simulink model "COSTEP"  (R2024b)
settings: Solver=FixedStepAuto  StartTime=0.0  StopTime=25  FixedStep=1/3600  RelTol=1e-3
model workspace (MAT data in the model file):
  AD : Simulink.Parameter (value not decoded)
  AG : Simulink.Parameter (value not decoded)
  AH : Simulink.Parameter (value not decoded)
  AV : Simulink.Parameter (value not decoded)
  AVP : Simulink.Parameter (value not decoded)
  BCHL : Simulink.Parameter (value not decoded)
  BCHV : Simulink.Parameter (value not decoded)
  BD : Simulink.Parameter (value not decoded)
  BDIST : Simulink.Parameter (value not decoded)
  BG : Simulink.Parameter (value not decoded)
  BH : Simulink.Parameter (value not decoded)
  BVP : Simulink.Parameter (value not decoded)
  CD : Simulink.Parameter (value not decoded)
  CDIST : Simulink.Parameter (value not decoded)
  CG : Simulink.Parameter (value not decoded)
  CH : Simulink.Parameter (value not decoded)
  CVP : Simulink.Parameter (value not decoded)
  DDIST : Simulink.Parameter (value not decoded)
  DIST_CONST : Simulink.Parameter (value not decoded)
  ISV : Simulink.Parameter (value not decoded)
  TLAST : Simulink.Parameter (value not decoded)
  TNEXT : Simulink.Parameter (value not decoded)
  XMW : Simulink.Parameter (value not decoded)
  XNS : Simulink.Parameter (value not decoded)
  XNS2 : Simulink.Parameter (value not decoded)
  XNS3 : Simulink.Parameter (value not decoded)
  XNSADD : Simulink.Parameter (value not decoded)
  XNSE : Simulink.Parameter (value not decoded)
symbols that are objects in the model workspace (value not decoded): AD, AG, AH, AV, AVP, BD, BG, BH, BVP, CD, CG, CH, CVP, XMW, XNS, XNS2, XNS3, XNSE
undefined symbols (not defined in the file or in its folder): magnitude, msgbox, SETPT, XMEAS, XMV
libraries: mylib x381, dspindex x31
(part 6 of 12)

== system COSTEP/Reactor/Holdup of Components in Reactor/Holdup of Vapour Components in Reactor ==
  YY(1:8) : Inport
  Bus Creator : BusCreator  Inputs=3
  Bus Selector : BusSelector  OutputSignals=YY(1),YY(2),YY(3)
  UCVR(1) Holdup of Component A (Vapour) in Reactor lb-mol : Gain
  UCVR(2) Holdup of Component B (Vapour) in Reactor lb-mol : Gain
  UCVR(3) Holdup of Component C (Vapour) in Reactor lb-mol : Gain
  UCVR : Outport  PortDimensions=3  VectorParamsAs1DForOutWhenUnconnected=off
  wires:
  UCVR(2) Holdup of Component B (Vapour) in Reactor lb-mol/1 -> Bus Creator/2  "UCVR(2)"
  Bus Selector/2 -> UCVR(2) Holdup of Component B (Vapour) in Reactor lb-mol/1  "<YY(2)>"
  Bus Selector/3 -> UCVR(3) Holdup of Component C (Vapour) in Reactor lb-mol/1  "<YY(3)>"
  UCVR(3) Holdup of Component C (Vapour) in Reactor lb-mol/1 -> Bus Creator/3  "UCVR(3)"
  UCVR(1) Holdup of Component A (Vapour) in Reactor lb-mol/1 -> Bus Creator/1  "UCVR(1)"
  Bus Creator/1 -> UCVR/1
  YY(1:8)/1 -> Bus Selector/1
  Bus Selector/1 -> UCVR(1) Holdup of Component A (Vapour) in Reactor lb-mol/1  "<YY(1)>"

== system COSTEP/Reactor/Holdup of Components in Reactor/Liquid Component Fraction in Reactor lb-mol ==
  UTLR : Inport
  UCLR : Inport  Port=2
  Bus Creator : BusCreator  Inputs=8
  Bus Selector : BusSelector  OutputSignals=UCLR(1),UCLR(2),UCLR(3),UCLR(4),UCLR(5),UCLR(6),UCLR(7),UCLR(8)
  XLR(1) : Product  Inputs=*/
  XLR(2) : Product  Inputs=*/
  XLR(3) : Product  Inputs=*/
  XLR(4) : Product  Inputs=*/
  XLR(5) : Product  Inputs=*/
  XLR(6) : Product  Inputs=*/
  XLR(7) : Product  Inputs=*/
  XLR(8) : Product  Inputs=*/
  XLR : Outport  VectorParamsAs1DForOutWhenUnconnected=off
  wires:
  XLR(5)/1 -> Bus Creator/5  "XLR(5)"
  Bus Selector/3 -> XLR(3)/1  "<UCLR(3)>"
  UTLR/1 -> XLR(8)/2, XLR(7)/2, XLR(6)/2, XLR(5)/2, XLR(4)/2, XLR(3)/2, XLR(2)/2, XLR(1)/2
  Bus Selector/7 -> XLR(7)/1  "<UCLR(7)>"
  XLR(8)/1 -> Bus Creator/8  "XLR(8)"
  XLR(7)/1 -> Bus Creator/7  "XLR(7)"
  Bus Selector/8 -> XLR(8)/1  "<UCLR(8)>"
  Bus Selector/5 -> XLR(5)/1  "<UCLR(5)>"
  Bus Selector/4 -> XLR(4)/1  "<UCLR(4)>"
  XLR(2)/1 -> Bus Creator/2  "XLR(2)"
  Bus Selector/6 -> XLR(6)/1  "<UCLR(6)>"
  XLR(3)/1 -> Bus Creator/3  "XLR(3)"
  UCLR/1 -> Bus Selector/1
  Bus Selector/1 -> XLR(1)/1  "<UCLR(1)>"
  XLR(4)/1 -> Bus Creator/4  "XLR(4)"
  Bus Selector/2 -> XLR(2)/1  "<UCLR(2)>"
  XLR(6)/1 -> Bus Creator/6  "XLR(6)"
  XLR(1)/1 -> Bus Creator/1  "XLR(1)"
  Bus Creator/1 -> XLR/1

== system COSTEP/Reactor/Holdup of Components in Reactor/Subsystem ==
  Properties of Stream 6 : Inport
  Bus Creator1 : BusCreator  Inputs=8
  Bus Selector1 : BusSelector  OutputSignals=FCM(I;6) = FCM(I;7)
  Multiport Selector : dspindex/Multiport Selector  rowsOrCols=Rows  idxCellArray={ 1,2,3,4,5,6,7,8}  idxErrMode=Clip Index
  FCM(I;7) : Outport  VectorParamsAs1DForOutWhenUnconnected=off
  wires:
  Multiport Selector/8 -> Bus Creator1/8  "FCM(8;7)"
  Multiport Selector/4 -> Bus Creator1/4  "FCM(4;7)"
  Multiport Selector/1 -> Bus Creator1/1  "FCM(1;7)"
  Bus Selector1/1 -> Multiport Selector/1  "<FCM(I;6) = FCM(I;7)>"
  Multiport Selector/6 -> Bus Creator1/6  "FCM(6;7)"
  Multiport Selector/2 -> Bus Creator1/2  "FCM(2;7)"
  Properties of Stream 6/1 -> Bus Selector1/1
  Multiport Selector/7 -> Bus Creator1/7  "FCM(7;7)"
  Multiport Selector/5 -> Bus Creator1/5  "FCM(5;7)"
  Multiport Selector/3 -> Bus Creator1/3  "FCM(3;7)"
  Bus Creator1/1 -> FCM(I;7)/1

== system COSTEP/Reactor/Holdup of Components in Reactor/Subsystem1 ==
  Bus Creator1 : BusCreator  Inputs=8
  Bus Selector2 : BusSelector  OutputSignals=signal1.FCM(I;8)
  Multiport Selector1 : dspindex/Multiport Selector  rowsOrCols=Rows  idxCellArray={ 1,2,3,4,5,6,7,8}  idxErrMode=Clip Index
  FCM(I;8) : Outport  VectorParamsAs1DForOutWhenUnconnected=off
  wires:
  Multiport Selector1/4 -> Bus Creator1/4  "FCM(4;8)"
  Multiport Selector1/5 -> Bus Creator1/5  "FCM(5;8)"
  Multiport Selector1/6 -> Bus Creator1/6  "FCM(6;8)"
  Multiport Selector1/3 -> Bus Creator1/3  "FCM(3;8)"
  Multiport Selector1/8 -> Bus Creator1/8  "FCM(8;8)"
  Bus Selector2/1 -> Multiport Selector1/1  "<FCM(I;8)>"
  Multiport Selector1/2 -> Bus Creator1/2  "FCM(2;8)"
  Multiport Selector1/7 -> Bus Creator1/7  "FCM(7;8)"
  Multiport Selector1/1 -> Bus Creator1/1  "FCM(1;8)"
  Bus Creator1/1 -> FCM(I;8)/1
  [PropertiesStream8] -> Bus Selector2/1

== system COSTEP/Reactor/Holdup of Components in Reactor/YP(1) ==
  FCM(1,7) : Inport
  CRXR(1) : Inport  Port=2
  FCM(1,8) : Inport  Port=3
  " YP(1)" : Sum  Inputs=+-+
  Bus Selector : BusSelector  OutputSignals=FCM(1;7)
  Bus Selector1 : BusSelector  OutputSignals=FCM(1;8)
  Bus Selector2 : BusSelector  OutputSignals=CRXR(1)
  Constant : Constant
  Initial state variable : mylib/Initial state variable
  Integration : mylib/Integration  SystemSampleTime=-1  VariantActivationTime=update diagram  AllowFlexibleInterface=on  Latency=0  AutoFrameSizeCalculation=off
  YY(1) : Outport  VectorParamsAs1DForOutWhenUnconnected=off
  wires:
  FCM(1,7)/1 -> Bus Selector/1
  Bus Selector/1 -> " YP(1)"/1  "<FCM(1;7)>"
  FCM(1,8)/1 -> Bus Selector1/1
  Bus Selector1/1 -> " YP(1)"/2  "<FCM(1;8)>"
  CRXR(1)/1 -> Bus Selector2/1
  Bus Selector2/1 -> " YP(1)"/3  "<CRXR(1)>"
  " YP(1)"/1 -> Integration/1
  Initial state variable/1 -> Integration/2
  Integration/1 -> YY(1)/1
  Constant/1 -> Initial state variable/1

== system COSTEP/Reactor/Holdup of Components in Reactor/YP(2) ==
  FCM(2,7) : Inport
  FCM(2,8) : Inport  Port=2
  Bus Selector : BusSelector  OutputSignals=FCM(2;7)
  Bus Selector1 : BusSelector  OutputSignals=FCM(2;8)
  Constant : Constant  Value=2
  Initial state variable : mylib/Initial state variable
  Integration : mylib/Integration  SystemSampleTime=-1  VariantActivationTime=update diagram  AllowFlexibleInterface=on  Latency=0  AutoFrameSizeCalculation=off
  "YP(2) " : Sum  Inputs=+-
  YY(2) : Outport  VectorParamsAs1DForOutWhenUnconnected=off
  wires:
  FCM(2,8)/1 -> Bus Selector1/1
  FCM(2,7)/1 -> Bus Selector/1
  Bus Selector/1 -> "YP(2) "/1  "<FCM(2;7)>"
  Bus Selector1/1 -> "YP(2) "/2  "<FCM(2;8)>"
  "YP(2) "/1 -> Integration/1
  Initial state variable/1 -> Integration/2
  Integration/1 -> YY(2)/1
  Constant/1 -> Initial state variable/1

== system COSTEP/Reactor/Holdup of Components in Reactor/YP(3) ==
  FCM(3,7) : Inport
  CRXR(3) : Inport  Port=2
  FCM(3,8) : Inport  Port=3
  " YP(3)" : Sum  Inputs=+-+
  Bus Selector : BusSelector  OutputSignals=CRXR(3)
  Bus Selector1 : BusSelector  OutputSignals=FCM(3;8)
  Bus Selector2 : BusSelector  OutputSignals=FCM(3;7)
  Constant : Constant  Value=3
  Initial state variable : mylib/Initial state variable
  Integration : mylib/Integration  SystemSampleTime=-1  VariantActivationTime=update diagram  AllowFlexibleInterface=on  Latency=0  AutoFrameSizeCalculation=off
  YY(3) : Outport  VectorParamsAs1DForOutWhenUnconnected=off
  wires:
  CRXR(3)/1 -> Bus Selector/1
  FCM(3,8)/1 -> Bus Selector1/1
  FCM(3,7)/1 -> Bus Selector2/1
  Bus Selector/1 -> " YP(3)"/3  "<CRXR(3)>"
  Bus Selector1/1 -> " YP(3)"/2  "<FCM(3;8)>"
  Bus Selector2/1 -> " YP(3)"/1  "<FCM(3;7)>"
  " YP(3)"/1 -> Integration/1
  Initial state variable/1 -> Integration/2
  Integration/1 -> YY(3)/1
  Constant/1 -> Initial state variable/1

== system COSTEP/Reactor/Holdup of Components in Reactor/YP(4) ==
  FCM(4,7) : Inport
  CRXR(4) : Inport  Port=2
  FCM(4,8) : Inport  Port=3
  " " : Sum  Inputs=+-+
  Bus Selector : BusSelector  OutputSignals=CRXR(4)
  Bus Selector1 : BusSelector  OutputSignals=FCM(4;8)
  Bus Selector2 : BusSelector  OutputSignals=FCM(4;7)
  Constant : Constant  Value=4
  Initial state variable : mylib/Initial state variable
  Integration : mylib/Integration  SystemSampleTime=-1  VariantActivationTime=update diagram  AllowFlexibleInterface=on  Latency=0  AutoFrameSizeCalculation=off
  "YY(4) " : Outport  VectorParamsAs1DForOutWhenUnconnected=off
  wires:
  CRXR(4)/1 -> Bus Selector/1
  FCM(4,8)/1 -> Bus Selector1/1
  FCM(4,7)/1 -> Bus Selector2/1
  Bus Selector/1 -> " "/3  "<CRXR(4)>"
  Bus Selector1/1 -> " "/2  "<FCM(4;8)>"
  Bus Selector2/1 -> " "/1  "<FCM(4;7)>"
  " "/1 -> Integration/1
  Initial state variable/1 -> Integration/2
  Integration/1 -> "YY(4) "/1
  Constant/1 -> Initial state variable/1

== system COSTEP/Reactor/Holdup of Components in Reactor/YP(5) ==
  FCM(5,7) : Inport
  CRXR(5) : Inport  Port=2
  FCM(5,8) : Inport  Port=3
  " " : Sum  Inputs=+-+
  Bus Selector : BusSelector  OutputSignals=CRXR(5)
  Bus Selector1 : BusSelector  OutputSignals=FCM(5;8)
  Bus Selector2 : BusSelector  OutputSignals=FCM(5;7)
  Constant : Constant  Value=5
  Initial state variable : mylib/Initial state variable
  Integration : mylib/Integration  SystemSampleTime=-1  VariantActivationTime=update diagram  AllowFlexibleInterface=on  Latency=0  AutoFrameSizeCalculation=off
  "YY(5) " : Outport  VectorParamsAs1DForOutWhenUnconnected=off
  wires:
  CRXR(5)/1 -> Bus Selector/1
  FCM(5,8)/1 -> Bus Selector1/1
  FCM(5,7)/1 -> Bus Selector2/1
  Bus Selector/1 -> " "/3  "<CRXR(5)>"
  Bus Selector1/1 -> " "/2  "<FCM(5;8)>"
  Bus Selector2/1 -> " "/1  "<FCM(5;7)>"
  " "/1 -> Integration/1
  Initial state variable/1 -> Integration/2
  Integration/1 -> "YY(5) "/1
  Constant/1 -> Initial state variable/1

== system COSTEP/Reactor/Holdup of Components in Reactor/YP(6) ==
  FCM(6,7) : Inport
  CRXR(6) : Inport  Port=2
  FCM(6,8) : Inport  Port=3
  " " : Sum  Inputs=+-+
  Bus Selector : BusSelector  OutputSignals=CRXR(6)
  Bus Selector1 : BusSelector  OutputSignals=FCM(6;8)
  Bus Selector2 : BusSelector  OutputSignals=FCM(6;7)
  Constant : Constant  Value=6
  Initial state variable : mylib/Initial state variable
  Integration : mylib/Integration  SystemSampleTime=-1  VariantActivationTime=update diagram  AllowFlexibleInterface=on  Latency=0  AutoFrameSizeCalculation=off
  "YY(6) " : Outport  VectorParamsAs1DForOutWhenUnconnected=off
  wires:
  CRXR(6)/1 -> Bus Selector/1
  FCM(6,8)/1 -> Bus Selector1/1
  FCM(6,7)/1 -> Bus Selector2/1
  Bus Selector/1 -> " "/3  "<CRXR(6)>"
  Bus Selector1/1 -> " "/2  "<FCM(6;8)>"
  Bus Selector2/1 -> " "/1  "<FCM(6;7)>"
  " "/1 -> Integration/1
  Initial state variable/1 -> Integration/2
  Integration/1 -> "YY(6) "/1
  Constant/1 -> Initial state variable/1

== system COSTEP/Reactor/Holdup of Components in Reactor/YP(7) ==
  FCM(7,7) : Inport
  CRXR(7) : Inport  Port=2
  FCM(7,8) : Inport  Port=3
  " " : Sum  Inputs=+-+
  Bus Selector : BusSelector  OutputSignals=CRXR(7)
  Bus Selector1 : BusSelector  OutputSignals=FCM(7;8)
  Bus Selector2 : BusSelector  OutputSignals=FCM(7;7)
  Constant : Constant  Value=7
  Initial state variable : mylib/Initial state variable
  Integration : mylib/Integration  SystemSampleTime=-1  VariantActivationTime=update diagram  AllowFlexibleInterface=on  Latency=0  AutoFrameSizeCalculation=off
  "YY(7) " : Outport  VectorParamsAs1DForOutWhenUnconnected=off
  wires:
  CRXR(7)/1 -> Bus Selector/1
  FCM(7,8)/1 -> Bus Selector1/1
  FCM(7,7)/1 -> Bus Selector2/1
  Bus Selector/1 -> " "/3  "<CRXR(7)>"
  Bus Selector1/1 -> " "/2  "<FCM(7;8)>"
  Bus Selector2/1 -> " "/1  "<FCM(7;7)>"
  " "/1 -> Integration/1
  Initial state variable/1 -> Integration/2
  Integration/1 -> "YY(7) "/1
  Constant/1 -> Initial state variable/1

== system COSTEP/Reactor/Holdup of Components in Reactor/YP(8) ==
  FCM(8,7) : Inport
  CRXR(8) : Inport  Port=2
  FCM(8,8) : Inport  Port=3
  " " : Sum  Inputs=+-+
  Bus Selector : BusSelector  OutputSignals=CRXR(8)
  Bus Selector1 : BusSelector  OutputSignals=FCM(8;8)
  Bus Selector2 : BusSelector  OutputSignals=FCM(8;7)
  Constant : Constant  Value=8
  Initial state variable : mylib/Initial state variable
  Integration : mylib/Integration  SystemSampleTime=-1  VariantActivationTime=update diagram  AllowFlexibleInterface=on  Latency=0  AutoFrameSizeCalculation=off
  "YY(8) " : Outport  VectorParamsAs1DForOutWhenUnconnected=off
  wires:
  CRXR(8)/1 -> Bus Selector/1
  FCM(8,8)/1 -> Bus Selector1/1
  FCM(8,7)/1 -> Bus Selector2/1
  Bus Selector/1 -> " "/3  "<CRXR(8)>"
  Bus Selector1/1 -> " "/2  "<FCM(8;8)>"
  Bus Selector2/1 -> " "/1  "<FCM(8;7)>"
  " "/1 -> Integration/1
  Initial state variable/1 -> Integration/2
  Integration/1 -> "YY(8) "/1
  Constant/1 -> Initial state variable/1

== system COSTEP/Reactor/Pressure of Reactor/Subsystem ==
  TKR : Inport
  VVR : Inport  Port=2
  UCVR : Inport  Port=3
  Bus Selector : BusSelector  OutputSignals=UCVR(1),UCVR(2),UCVR(3)
  PPR(1) Partial pressure of Component A mmHg : Product  Inputs=***/
  PPR(2) Partial pressure of Component B mmHg : Product  Inputs=***/
  PPR(3) Partial pressure of Component C mmHg : Product  Inputs=***/
  RG Universal Gas Constant ft³·mmHg/K·lb-mol : Constant  Value=998.9
  PPR(1) : Outport  VectorParamsAs1DForOutWhenUnconnected=off
  PPR(2) : Outport  Port=2  VectorParamsAs1DForOutWhenUnconnected=off
  PPR(3) : Outport  Port=3  VectorParamsAs1DForOutWhenUnconnected=off
  wires:
  Bus Selector/2 -> PPR(2) Partial pressure of Component B mmHg/1  "<UCVR(2)>"
  TKR/1 -> PPR(3) Partial pressure of Component C mmHg/3, PPR(2) Partial pressure of Component B mmHg/3, PPR(1) Partial pressure of Component A mmHg/3
  VVR/1 -> PPR(3) Partial pressure of Component C mmHg/4, PPR(2) Partial pressure of Component B mmHg/4, PPR(1) Partial pressure of Component A mmHg/4
  RG Universal Gas Constant ft³·mmHg/K·lb-mol/1 -> PPR(3) Partial pressure of Component C mmHg/2, PPR(1) Partial pressure of Component A mmHg/2, PPR(2) Partial pressure of Component B mmHg/2
  PPR(2) Partial pressure of Component B mmHg/1 -> PPR(2)/1  "PPR(2)"
  Bus Selector/1 -> PPR(1) Partial pressure of Component A mmHg/1  "<UCVR(1)>"
  Bus Selector/3 -> PPR(3) Partial pressure of Component C mmHg/1  "<UCVR(3)>"
  PPR(1) Partial pressure of Component A mmHg/1 -> PPR(1)/1  "PPR(1)"
  PPR(3) Partial pressure of Component C mmHg/1 -> PPR(3)/1  "PPR(3)"
  UCVR/1 -> Bus Selector/1

== system COSTEP/Reactor/Pressure of Reactor/VPR Vapour Pressure mmHg ==
  TCR : Inport
  AVP(I) Antoine Coefficient A ln(mmHg) : Constant  Value=AVP
  Add : Sum
  Add1 : Sum
  BVP(I) Antoine Coefficient B ln(mmHg)·°C : Constant  Value=BVP
  CVP(I) Antoine Coefficient C °C : Constant  Value=CVP
  Divide : Product  Inputs=*/
  Math Function : Math  SignedPower=on
  VPR : Outport  VectorParamsAs1DForOutWhenUnconnected=off
  wires:
  BVP(I) Antoine Coefficient B ln(mmHg)·°C/1 -> Divide/1
  CVP(I) Antoine Coefficient C °C/1 -> Add/1
  AVP(I) Antoine Coefficient A ln(mmHg)/1 -> Add1/1
  Add/1 -> Divide/2
  Divide/1 -> Add1/2
  Add1/1 -> Math Function/1
  Math Function/1 -> VPR/1
  TCR/1 -> Add/2

== system COSTEP/Reactor/Reaction Rates/Component reaction rate lb-mol//h ==
  RR : Inport
  Bus Creator : BusCreator  Inputs=7
  Subsystem : Subsystem
  Subsystem1 : Subsystem
  Subsystem2 : Subsystem
  Subsystem3 : Subsystem
  Subsystem4 : Subsystem
  Subsystem5 : Subsystem
  Subsystem6 : Subsystem
  CRXR : Outport  VectorParamsAs1DForOutWhenUnconnected=off
  wires:
  RR/1 -> Subsystem4/1(RR), Subsystem6/1(RR), Subsystem5/1(RR), Subsystem3/1(RR), Subsystem1/1(RR), Subsystem/1(RR), Subsystem2/1(RR)
  Bus Creator/1 -> CRXR/1
  Subsystem/1(CRXR(1)) -> Bus Creator/1
  Subsystem1/1(CRXR(3)) -> Bus Creator/2
  Subsystem2/1(CRXR(4)) -> Bus Creator/3
  Subsystem3/1(CRXR(5)) -> Bus Creator/4
  Subsystem4/1(CRXR(6)) -> Bus Creator/5
  Subsystem5/1(CRXR(7)) -> Bus Creator/6
  Subsystem6/1(CRXR(8)) -> Bus Creator/7

== system COSTEP/Reactor/Reaction Rates/Reaction Heat MBtu//h ==
  RR : Inport
  Bus Selector : BusSelector  OutputSignals=RR(1),RR(2)
  HTR(1) Heat of Reaction 1 MBtu/lb-mol : Constant  Value=0.06899381054
  HTR(2) Heat of reaction 2 MBtu/lb-mol : Constant  Value=0.05
  Product : Product
  Product1 : Product
  RH Total reaction heat MBtu/h : Sum
  RH : Outport  VectorParamsAs1DForOutWhenUnconnected=off
  wires:
  HTR(2) Heat of reaction 2 MBtu/lb-mol/1 -> Product1/2
  Product/1 -> RH Total reaction heat MBtu/h/1
  Product1/1 -> RH Total reaction heat MBtu/h/2
  HTR(1) Heat of Reaction 1 MBtu/lb-mol/1 -> Product/2
  RH Total reaction heat MBtu/h/1 -> RH/1
  RR/1 -> Bus Selector/1
  Bus Selector/1 -> Product/1  "<RR(1)>"
  Bus Selector/2 -> Product1/1  "<RR(2)>"

== system COSTEP/Reactor/Reaction Rates/Reaction rates lb-mol//h ==
  TKR : Inport
  PPR : Inport  Port=2
  VVR : Inport  Port=3
  " Reaction rate of reaction 4 lb-mol/ft3·h    " : Subsystem
  Bus Creator : BusCreator  Inputs=4
  Product{,1..3} (4 alike) : Product
  Reaction rate of reaction 1 lb-mol/ft3·h : Subsystem
  Reaction rate of reaction 2 lb-mol/ft3·h : Subsystem
  "Reaction rate of reaction 3 lb-mol/ft3·h  " : Subsystem
  RR : Outport  VectorParamsAs1DForOutWhenUnconnected=off
  wires:
  TKR/1 -> Reaction rate of reaction 1 lb-mol/ft3·h/2(TKR), " Reaction rate of reaction 4 lb-mol/ft3·h    "/2(TKR), "Reaction rate of reaction 3 lb-mol/ft3·h  "/2(TKR), Reaction rate of reaction 2 lb-mol/ft3·h/2(TKR)
  PPR/1 -> Reaction rate of reaction 1 lb-mol/ft3·h/1(PPR), " Reaction rate of reaction 4 lb-mol/ft3·h    "/1(PPR), "Reaction rate of reaction 3 lb-mol/ft3·h  "/1(PPR), Reaction rate of reaction 2 lb-mol/ft3·h/1(PPR)
  Bus Creator/1 -> RR/1
  Reaction rate of reaction 1 lb-mol/ft3·h/1(RR(1)) -> Product/1  "RR(1)"
  VVR/1 -> Product/2, Product3/2, Product2/2, Product1/2
  Product/1 -> Bus Creator/1  "RR(1)"
  Reaction rate of reaction 2 lb-mol/ft3·h/1(RR(2)) -> Product1/1  "RR(2)"
  Product1/1 -> Bus Creator/2  "RR(2)"
  "Reaction rate of reaction 3 lb-mol/ft3·h  "/1(RR(3)) -> Product2/1  "RR(3)"
  Product2/1 -> Bus Creator/3  "RR(3)"
  " Reaction rate of reaction 4 lb-mol/ft3·h    "/1(RR(4)) -> Product3/1  "RR(4)"
  Product3/1 -> Bus Creator/4  "RR(4)"

== system COSTEP/Reactor/Reactor Heat exchanger/Position of Valve 10 % ==
  Bus Selector : BusSelector  OutputSignals=XMV(10)
  Bus Selector1 : BusSelector  OutputSignals=IDV(14)
  Constant : Constant  Value=48
  Control valve : mylib/Control valve  SystemSampleTime=-1  VariantActivationTime=update diagram  AllowFlexibleInterface=on  Latency=0  AutoFrameSizeCalculation=off
  Divide : Product  Inputs=*/
  Initial state variable : mylib/Initial state variable
  Integration : mylib/Integration  SystemSampleTime=-1  VariantActivationTime=update diagram  AllowFlexibleInterface=on  Latency=0  AutoFrameSizeCalculation=off
  Subtract : Sum  Inputs=+-
  VTAU(10) : Constant  Value=5/3600
  "YY(48) " : Outport  PortDimensions=1  VectorParamsAs1DForOutWhenUnconnected=off
  wires:
  Subtract/1 -> Divide/1
  Control valve/1 -> Subtract/1
  VTAU(10)/1 -> Divide/2
  Divide/1 -> Integration/1
  [XMV] -> Bus Selector/1
  Bus Selector/1 -> Control valve/1  "<XMV(10)>"
  [IDV] -> Bus Selector1/1
  Bus Selector1/1 -> Control valve/2  "<IDV(14)>"
  Initial state variable/1 -> Integration/2
  Integration/1 -> Subtract/2, "YY(48) "/1
  Constant/1 -> Initial state variable/1

== system COSTEP/Reactor/Reactor Heat exchanger/Position of Valve 12 % ==
  Bus Selector : BusSelector  OutputSignals=XMV(12)
  Constant : Constant  Value=50
  Control valve : Subsystem
  Divide : Product  Inputs=*/
  Initial state variable : mylib/Initial state variable
  Integration : mylib/Integration  SystemSampleTime=-1  VariantActivationTime=update diagram  AllowFlexibleInterface=on  Latency=0  AutoFrameSizeCalculation=off
  Subtract : Sum  Inputs=+-
  VTAU(12) : Constant  Value=5/3600
  "YY(50) " : Outport  PortDimensions=1  VectorParamsAs1DForOutWhenUnconnected=off
  wires:
  Integration/1 -> "YY(50) "/1, Subtract/2  "VPOS(12)"
  Subtract/1 -> Divide/1
  Control valve/1(VCV(12)) -> Subtract/1
  VTAU(12)/1 -> Divide/2
  Divide/1 -> Integration/1
  Initial state variable/1 -> Integration/2
  [XMV] -> Bus Selector/1
  Bus Selector/1 -> Control valve/1(XMV(12))  "<XMV(12)>"
  Constant/1 -> Initial state variable/1

== system COSTEP/Reactor/Reactor Heat exchanger/Reactor Heat exchanger ==
  VLR : Inport
  VPOS(10) : Inport  Port=2
  VRNG(10) : Inport  Port=3
  VPOS(12) : Inport  Port=4
  TCR : Inport  Port=5
  AGSP Agitation speed : Subsystem
  Cooling water outlet temperature : Subsystem
  FWR Flow of cooling water to reactor gallons per minute : Subsystem
  Subsystem : Subsystem
  Subsystem2 : Subsystem
  Subsystem3 : Subsystem
  "QUR " : Outport  PortDimensions=1  VectorParamsAs1DForOutWhenUnconnected=off
  tag scope: FWR=global
  wires:
  VRNG(10)/1 -> FWR Flow of cooling water to reactor gallons per minute/2(VRNG(10))
  VLR/1 -> Subsystem/1(VLR)
  VPOS(10)/1 -> FWR Flow of cooling water to reactor gallons per minute/1(VPOS(10))
  VPOS(12)/1 -> AGSP Agitation speed/1(VPOS(12))
  FWR Flow of cooling water to reactor gallons per minute/1(FWR) -> [FWR], Cooling water outlet temperature/1(FWR)
  Subsystem/1("UARLEV ") -> Subsystem2/1(UARLEV)
  AGSP Agitation speed/1(AGSP) -> Subsystem2/2(AGSP)
  Subsystem3/1("QUR ") -> Cooling water outlet temperature/2(QUR), "QUR "/1
  Subsystem2/1("UAR ") -> Subsystem3/1(UAR)
  Cooling water outlet temperature/1("YY(37) ") -> Subsystem3/2(TWR)
  TCR/1 -> Subsystem3/3(TCR)

== system COSTEP/Reactor/Reactor Heat exchanger/VRNG(10) Max flow of water through valve Gallons per minute ==
  Bus Selector : BusSelector  OutputSignals=signal3.TESUB8(19)
  VRNG(10) : Outport  PortDimensions=1  VectorParamsAs1DForOutWhenUnconnected=off
  wires:
  [TESUB8] -> Bus Selector/1
  Bus Selector/1 -> VRNG(10)/1  "<TESUB8(19)>"

== system COSTEP/Reactor/Stream 8/HST(8) Molar Enthalpy of Stream 8 MBtu//lb-mol ==
  ITY : Inport
  T : Inport  Port=2
  XST(I,I) : Inport  Port=3
  "Enthalpy of Stream " : mylib/Enthalpy of Stream   SystemSampleTime=-1  VariantActivationTime=update diagram  AllowFlexibleInterface=on  Latency=0  AutoFrameSizeCalculation=off
  "H " : Outport  VectorParamsAs1DForOutWhenUnconnected=off
  wires:
  ITY/1 -> "Enthalpy of Stream "/1
  T/1 -> "Enthalpy of Stream "/2
  XST(I,I)/1 -> "Enthalpy of Stream "/3
  "Enthalpy of Stream "/1 -> "H "/1

== system COSTEP/Reactor/Stream 8/Subsystem ==
  Abs : Abs  SaturateOnIntegerOverflow=off
  Bus Selector : BusSelector  OutputSignals=signal2.TESUB8(12)
  Constant : Constant  Value=0.0
  Constant1 : Constant  Value=4574.21
  Constant2 : Constant
  Constant3 : Constant  Value=0.25
  DLP : Sum  Inputs=+-
  DLP Pressure drop between separator and reactor : Merge
  FLMS : Product  Inputs=3
  If : If  IfExpression=u1 < 0
  If Action Subsystem : Subsystem  TreatAsAtomicUnit=on
  If Action Subsystem1 : Subsystem  TreatAsAtomicUnit=on
  Product : Product
  Sqrt : Sqrt
  Subtract : Sum  Inputs=+-
  "FLMS " : Outport  VectorParamsAs1DForOutWhenUnconnected=off
  wires:
  [PTS] -> DLP/2
  If Action Subsystem/1(Out1) -> DLP Pressure drop between separator and reactor/1
  Constant2/1 -> Subtract/1
  DLP/1 -> If/1, If Action Subsystem1/1(In1)
  DLP Pressure drop between separator and reactor/1 -> Abs/1
  If Action Subsystem1/1(Out1) -> DLP Pressure drop between separator and reactor/2
  If/1 -> If Action Subsystem/Action
  Sqrt/1 -> FLMS/2
  [PTR] -> DLP/1
  Abs/1 -> Sqrt/1
  Constant3/1 -> Product/1
  Constant1/1 -> FLMS/1
  [TESUB8] -> Bus Selector/1
  Subtract/1 -> FLMS/3
  Bus Selector/1 -> Product/2  "<TESUB8(12)>"
  If/2 -> If Action Subsystem1/Action
  Product/1 -> Subtract/2
  Constant/1 -> If Action Subsystem/1(In1)
  FLMS/1 -> "FLMS "/1

== system COSTEP/Reactor/Stream 8/XMWS(8) Molecular weight of Stream 8 lb//lb-mol ==
  XST(I,8) : Inport
  Product : Product
  Sum of Elements : Sum  Inputs=+
  "XMW(I) Molecular weight of components lb/lb-mol " : Constant  Value=[2;25.4;28;32;46;48;62;76]
  XMWS(8) : Outport  VectorParamsAs1DForOutWhenUnconnected=off
  wires:
  Sum of Elements/1 -> XMWS(8)/1
  Product/1 -> Sum of Elements/1
  XST(I,8)/1 -> Product/1
  "XMW(I) Molecular weight of components lb/lb-mol "/1 -> Product/2

== system COSTEP/Reactor/Volume of Reactor/DLR Molar Density of Liquids in Reactor lb-mol//ft³     ==
  XLR : Inport
  TCR : Inport  Port=2
  "DLR Molar Density of Liquids in Reactor lb-mol/ft³ " : Subsystem
  "DLR " : Outport  VectorParamsAs1DForOutWhenUnconnected=off
  wires:
  "DLR Molar Density of Liquids in Reactor lb-mol/ft³ "/1("R ") -> "DLR "/1
  TCR/1 -> "DLR Molar Density of Liquids in Reactor lb-mol/ft³ "/2(T)
  XLR/1 -> "DLR Molar Density of Liquids in Reactor lb-mol/ft³ "/1(X)

== system COSTEP/Separator/Holdup of Components in Separator/Holdup of Liquid Components in Separator ==
  YY(10:17) : Inport
  Bus Creator : BusCreator  Inputs=8
  Bus Selector : BusSelector  OutputSignals=YY(13),YY(14),YY(15),YY(16),YY(17)
  UCLS(1) Holdup of Component A (Liquid) in Separator lb-mol : Constant  Value=0
  UCLS(2) Holdup of Component B (Liquid) in Separator lb-mol : Constant  Value=0
  UCLS(4) Holdup of Component D (Liquid) in Separator lb-mol : Gain
  UCLS(5) Holdup of Component E (Liquid) in Separator lb-mol : Gain
  UCLS(6) Holdup of Component F (Liquid) in Separator lb-mol : Gain
  UCLS(7) Holdup of Component G (Liquid) in Separator lb-mol : Gain
  UCLS(8) Holdup of Component H (Liquid) in Separator lb-mol : Gain
  UCLS3) Holdup of Component C (Liquid) in Separator lb-mol : Constant  Value=0
  UCLS : Outport  VectorParamsAs1DForOutWhenUnconnected=off
  wires:
  UCLS(2) Holdup of Component B (Liquid) in Separator lb-mol/1 -> Bus Creator/2  "UCLS(2)"
  UCLS(8) Holdup of Component H (Liquid) in Separator lb-mol/1 -> Bus Creator/8  "UCLS(8)"
  UCLS(1) Holdup of Component A (Liquid) in Separator lb-mol/1 -> Bus Creator/1  "UCLS(1)"
  UCLS(5) Holdup of Component E (Liquid) in Separator lb-mol/1 -> Bus Creator/5  "UCLS(5)"
  UCLS(4) Holdup of Component D (Liquid) in Separator lb-mol/1 -> Bus Creator/4  "UCLS(4)"
  UCLS3) Holdup of Component C (Liquid) in Separator lb-mol/1 -> Bus Creator/3  "UCLS(3)"
  UCLS(6) Holdup of Component F (Liquid) in Separator lb-mol/1 -> Bus Creator/6  "UCLS(6)"
  UCLS(7) Holdup of Component G (Liquid) in Separator lb-mol/1 -> Bus Creator/7  "UCLS(7)"
  YY(10:17)/1 -> Bus Selector/1
  Bus Creator/1 -> UCLS/1
  Bus Selector/1 -> UCLS(4) Holdup of Component D (Liquid) in Separator lb-mol/1  "<YY(13)>"
  Bus Selector/2 -> UCLS(5) Holdup of Component E (Liquid) in Separator lb-mol/1  "<YY(14)>"
  Bus Selector/3 -> UCLS(6) Holdup of Component F (Liquid) in Separator lb-mol/1  "<YY(15)>"
  Bus Selector/4 -> UCLS(7) Holdup of Component G (Liquid) in Separator lb-mol/1  "<YY(16)>"
  Bus Selector/5 -> UCLS(8) Holdup of Component H (Liquid) in Separator lb-mol/1  "<YY(17)>"

== system COSTEP/Separator/Holdup of Components in Separator/Holdup of Vapour Components in Separator ==
  YY(10:17) : Inport
  Bus Creator : BusCreator  Inputs=3
  Bus Selector : BusSelector  OutputSignals=YY(10),YY(11),YY(12)
  UCVS(1) Holdup of Component A (Vapour) in Separator lb-mol : Gain
  UCVS(2) Holdup of Component B (Vapour) in Separator lb-mol : Gain
  UCVS(3) Holdup of Component C (Vapour) in Separator lb-mol : Gain
  UCVS : Outport  VectorParamsAs1DForOutWhenUnconnected=off
  wires:
  UCVS(1) Holdup of Component A (Vapour) in Separator lb-mol/1 -> Bus Creator/1  "UCVS(1)"
  Bus Selector/3 -> UCVS(3) Holdup of Component C (Vapour) in Separator lb-mol/1  "<YY(12)>"
  UCVS(2) Holdup of Component B (Vapour) in Separator lb-mol/1 -> Bus Creator/2  "UCVS(2)"
  UCVS(3) Holdup of Component C (Vapour) in Separator lb-mol/1 -> Bus Creator/3  "UCVS(3)"
  Bus Creator/1 -> UCVS/1
  YY(10:17)/1 -> Bus Selector/1
  Bus Selector/1 -> UCVS(1) Holdup of Component A (Vapour) in Separator lb-mol/1  "<YY(10)>"
  Bus Selector/2 -> UCVS(2) Holdup of Component B (Vapour) in Separator lb-mol/1  "<YY(11)>"

== system COSTEP/Separator/Holdup of Components in Separator/Liquid Component Fraction in Separator ==
  UTLS : Inport
  UCLS : Inport  Port=2
  Bus Creator : BusCreator  Inputs=8
  Bus Selector : BusSelector  OutputSignals=UCLS(1),UCLS(2),UCLS(3),UCLS(4),UCLS(5),UCLS(6),UCLS(7),UCLS(8)
  XLS(1) : Product  Inputs=*/
  XLS(2) : Product  Inputs=*/
  XLS(3) : Product  Inputs=*/
  XLS(4) : Product  Inputs=*/
  XLS(5) : Product  Inputs=*/
  XLS(6) : Product  Inputs=*/
  XLS(7) : Product  Inputs=*/
  XLS(8) : Product  Inputs=*/
  XLS : Outport  VectorParamsAs1DForOutWhenUnconnected=off
  wires:
  Bus Selector/1 -> XLS(1)/1  "<UCLS(1)>"
  XLS(2)/1 -> Bus Creator/2  "XLS(2)"
  Bus Selector/7 -> XLS(7)/1  "<UCLS(7)>"
  XLS(3)/1 -> Bus Creator/3  "XLS(3)"
  Bus Selector/8 -> XLS(8)/1  "<UCLS(8)>"
  Bus Selector/3 -> XLS(3)/1  "<UCLS(3)>"
  XLS(7)/1 -> Bus Creator/7  "XLS(7)"
  XLS(1)/1 -> Bus Creator/1  "XLS(1)"
  Bus Selector/2 -> XLS(2)/1  "<UCLS(2)>"
  Bus Selector/5 -> XLS(5)/1  "<UCLS(5)>"
  Bus Selector/4 -> XLS(4)/1  "<UCLS(4)>"
  XLS(6)/1 -> Bus Creator/6  "XLS(6)"
  XLS(4)/1 -> Bus Creator/4  "XLS(4)"
  XLS(5)/1 -> Bus Creator/5  "XLS(5)"
  XLS(8)/1 -> Bus Creator/8  "XLS(8)"
  Bus Selector/6 -> XLS(6)/1  "<UCLS(6)>"
  Bus Creator/1 -> XLS/1
  UTLS/1 -> XLS(8)/2, XLS(7)/2, XLS(6)/2, XLS(5)/2, XLS(4)/2, XLS(3)/2, XLS(2)/2, XLS(1)/2
  UCLS/1 -> Bus Selector/1

== system COSTEP/Separator/Holdup of Components in Separator/Subsystem ==
  Properties of Stream 8 : Inport
  Bus Creator : BusCreator  Inputs=8
  Bus Selector : BusSelector  OutputSignals=FCM(I;8)
  FCM(1,8) : Gain
  FCM(2,8) : Gain
  FCM(3,8) : Gain
  FCM(4,8) : Gain
  FCM(5,8) : Gain
  FCM(6,8) : Gain
  FCM(7,8) : Gain
  FCM(8,8) : Gain
  Multiport Selector : dspindex/Multiport Selector  rowsOrCols=Rows  idxCellArray={ 1,2,3,4,5,6,7,8}  idxErrMode=Clip Index
  FCM(I;8) : Outport  VectorParamsAs1DForOutWhenUnconnected=off
  wires:
  Multiport Selector/3 -> FCM(3,8)/1
  Multiport Selector/6 -> FCM(6,8)/1
  Multiport Selector/8 -> FCM(8,8)/1
  Multiport Selector/2 -> FCM(2,8)/1
  Multiport Selector/7 -> FCM(7,8)/1
  Properties of Stream 8/1 -> Bus Selector/1
  Multiport Selector/4 -> FCM(4,8)/1
  Multiport Selector/1 -> FCM(1,8)/1
  Multiport Selector/5 -> FCM(5,8)/1
  Bus Selector/1 -> Multiport Selector/1  "<FCM(I;8)>"
  FCM(1,8)/1 -> Bus Creator/1  "FCM(1;8)"
  FCM(2,8)/1 -> Bus Creator/2  "FCM(2;8)"
  FCM(3,8)/1 -> Bus Creator/3  "FCM(3;8)"
  FCM(4,8)/1 -> Bus Creator/4  "FCM(4;8)"
  FCM(5,8)/1 -> Bus Creator/5  "FCM(5;8)"
  FCM(6,8)/1 -> Bus Creator/6  "FCM(6;8)"
  FCM(7,8)/1 -> Bus Creator/7  "FCM(7;8)"
  FCM(8,8)/1 -> Bus Creator/8  "FCM(8;8)"
  Bus Creator/1 -> FCM(I;8)/1

== system COSTEP/Separator/Holdup of Components in Separator/Subsystem1 ==
  Bus Creator : BusCreator  Inputs=8
  Bus Selector1 : BusSelector  OutputSignals=signal2.FCM(I;9)
  FCM(1,9) : Gain
  FCM(2,9) : Gain
  FCM(3,9) : Gain
  FCM(4,9) : Gain
  FCM(5,9) : Gain
  FCM(6,9) : Gain
  FCM(7,9) : Gain
  FCM(8,9) : Gain
  Multiport Selector1 : dspindex/Multiport Selector  rowsOrCols=Rows  idxCellArray={ 1,2,3,4,5,6,7,8}  idxErrMode=Clip Index
  FCM(I;9) : Outport  VectorParamsAs1DForOutWhenUnconnected=off
  wires:
  [PropertiesStream9] -> Bus Selector1/1
  Multiport Selector1/4 -> FCM(4,9)/1
  Bus Selector1/1 -> Multiport Selector1/1  "<FCM(I;9)>"
  Multiport Selector1/7 -> FCM(7,9)/1
  Multiport Selector1/3 -> FCM(3,9)/1
  Multiport Selector1/8 -> FCM(8,9)/1
  Multiport Selector1/6 -> FCM(6,9)/1
  Multiport Selector1/5 -> FCM(5,9)/1
  Multiport Selector1/2 -> FCM(2,9)/1
  Multiport Selector1/1 -> FCM(1,9)/1
  FCM(1,9)/1 -> Bus Creator/1  "FCM(1;9)"
  FCM(2,9)/1 -> Bus Creator/2  "FCM(2;9)"
  FCM(3,9)/1 -> Bus Creator/3  "FCM(3;9)"
  FCM(4,9)/1 -> Bus Creator/4  "FCM(4;9)"
  FCM(5,9)/1 -> Bus Creator/5  "FCM(5;9)"
  FCM(7,9)/1 -> Bus Creator/7  "FCM(7;9)"
  FCM(8,9)/1 -> Bus Creator/8  "FCM(8;9)"
  FCM(6,9)/1 -> Bus Creator/6  "FCM(6;9)"
  Bus Creator/1 -> FCM(I;9)/1

== system COSTEP/Separator/Holdup of Components in Separator/Subsystem2 ==
  Bus Creator : BusCreator  Inputs=8
  Bus Selector2 : BusSelector  OutputSignals=signal1.FCM(I;10)
  FCM(1,10) : Gain
  FCM(2,10) : Gain
  FCM(3,10) : Gain
  FCM(4,10) : Gain
  FCM(5,10) : Gain
  FCM(6,10) : Gain
  FCM(7,10) : Gain
  FCM(8,10) : Gain
  Multiport Selector2 : dspindex/Multiport Selector  rowsOrCols=Rows  idxCellArray={ 1,2,3,4,5,6,7,8}  idxErrMode=Clip Index
  FCM(I;10) : Outport  VectorParamsAs1DForOutWhenUnconnected=off
  wires:
  [PropertiesStream10] -> Bus Selector2/1
  FCM(4,10)/1 -> Bus Creator/4  "FCM(4;10)"
  Multiport Selector2/5 -> FCM(5,10)/1
  Multiport Selector2/4 -> FCM(4,10)/1
  FCM(2,10)/1 -> Bus Creator/2  "FCM(2;10)"
  Multiport Selector2/8 -> FCM(8,10)/1
  Multiport Selector2/7 -> FCM(7,10)/1
  FCM(8,10)/1 -> Bus Creator/8  "FCM(8;10)"
  Multiport Selector2/2 -> FCM(2,10)/1
  Multiport Selector2/3 -> FCM(3,10)/1
  Multiport Selector2/1 -> FCM(1,10)/1
  Bus Selector2/1 -> Multiport Selector2/1  "<FCM(I;10)>"
  Multiport Selector2/6 -> FCM(6,10)/1
  FCM(5,10)/1 -> Bus Creator/5  "FCM(5;10)"
  FCM(3,10)/1 -> Bus Creator/3  "FCM(3;10)"
  FCM(1,10)/1 -> Bus Creator/1  "FCM(1;10)"
  FCM(6,10)/1 -> Bus Creator/6  "FCM(6;10)"
  FCM(7,10)/1 -> Bus Creator/7  "FCM(7;10)"
  Bus Creator/1 -> FCM(I;10)/1

== system COSTEP/Separator/Holdup of Components in Separator/Subsystem3 ==
  Bus Creator : BusCreator  Inputs=8
  Bus Selector3 : BusSelector  OutputSignals=signal1.FCM(I;11)
  FCM(1,11) : Gain
  FCM(2,11) : Gain
  FCM(3,11) : Gain
  FCM(4,11) : Gain
  FCM(5,11) : Gain
  FCM(6,11) : Gain
  FCM(7,11) : Gain
  FCM(8,11) : Gain
  Multiport Selector3 : dspindex/Multiport Selector  rowsOrCols=Rows  idxCellArray={1,2,3,4,5,6,7,8}  idxErrMode=Clip Index
  FCM(I;11) : Outport  VectorParamsAs1DForOutWhenUnconnected=off
  wires:
  Multiport Selector3/3 -> FCM(3,11)/1
  Multiport Selector3/2 -> FCM(2,11)/1
  Multiport Selector3/5 -> FCM(5,11)/1
  Multiport Selector3/8 -> FCM(8,11)/1
  Bus Selector3/1 -> Multiport Selector3/1  "<FCM(I;11)>"
  Multiport Selector3/7 -> FCM(7,11)/1
  Multiport Selector3/6 -> FCM(6,11)/1
  Multiport Selector3/1 -> FCM(1,11)/1
  Multiport Selector3/4 -> FCM(4,11)/1
  [PropertiesStream11] -> Bus Selector3/1
  FCM(5,11)/1 -> Bus Creator/5  "FCM(5;11)"
  FCM(8,11)/1 -> Bus Creator/8  "FCM(8;11)"
  FCM(7,11)/1 -> Bus Creator/7  "FCM(7;11)"
  FCM(6,11)/1 -> Bus Creator/6  "FCM(6;11)"
  FCM(2,11)/1 -> Bus Creator/2  "FCM(2;11)"
  FCM(3,11)/1 -> Bus Creator/3  "FCM(3;11)"
  FCM(4,11)/1 -> Bus Creator/4  "FCM(4;11)"
  FCM(1,11)/1 -> Bus Creator/1  "FCM(1;11)"
  Bus Creator/1 -> FCM(I;11)/1

== system COSTEP/Separator/Holdup of Components in Separator/YP(10) ==
  FCM(1,8) : Inport
  FCM(1,9) : Inport  Port=2
  FCM(1,10) : Inport  Port=3
  FCM(1,11) : Inport  Port=4
  " " : Sum  Inputs=+---
  Bus Selector : BusSelector  OutputSignals=FCM(1;8)
  Bus Selector1 : BusSelector  OutputSignals=FCM(1;9)
  Bus Selector2 : BusSelector  OutputSignals=FCM(1;10)
  Bus Selector3 : BusSelector  OutputSignals=FCM(1;11)
  Constant : Constant  Value=10
  Initial state variable : mylib/Initial state variable
  Integration : mylib/Integration  SystemSampleTime=-1  VariantActivationTime=update diagram  AllowFlexibleInterface=on  Latency=0  AutoFrameSizeCalculation=off
  YY(10) : Outport  VectorParamsAs1DForOutWhenUnconnected=off
  wires:
  Initial state variable/1 -> Integration/2
  FCM(1,10)/1 -> Bus Selector2/1
  FCM(1,9)/1 -> Bus Selector1/1
  FCM(1,8)/1 -> Bus Selector/1
  " "/1 -> Integration/1
  Integration/1 -> YY(10)/1
  FCM(1,11)/1 -> Bus Selector3/1
  Bus Selector/1 -> " "/1  "<FCM(1;8)>"
  Bus Selector1/1 -> " "/2  "<FCM(1;9)>"
  Bus Selector2/1 -> " "/3  "<FCM(1;10)>"
  Bus Selector3/1 -> " "/4  "<FCM(1;11)>"
  Constant/1 -> Initial state variable/1

== system COSTEP/Separator/Holdup of Components in Separator/YP(11) ==
  FCM(2,8) : Inport
  FCM(2,9) : Inport  Port=2
  FCM(2,10) : Inport  Port=3
  FCM(2,11) : Inport  Port=4
  " " : Sum  Inputs=+---
  Bus Selector : BusSelector  OutputSignals=FCM(2;8)
  Bus Selector1 : BusSelector  OutputSignals=FCM(2;9)
  Bus Selector2 : BusSelector  OutputSignals=FCM(2;10)
  Bus Selector3 : BusSelector  OutputSignals=FCM(2;11)
  Constant : Constant  Value=11
  Initial state variable : mylib/Initial state variable
  Integration : mylib/Integration  SystemSampleTime=-1  VariantActivationTime=update diagram  AllowFlexibleInterface=on  Latency=0  AutoFrameSizeCalculation=off
  YY(11) : Outport  VectorParamsAs1DForOutWhenUnconnected=off
  wires:
  Integration/1 -> YY(11)/1
  FCM(2,8)/1 -> Bus Selector/1
  FCM(2,9)/1 -> Bus Selector1/1
  FCM(2,10)/1 -> Bus Selector2/1
  FCM(2,11)/1 -> Bus Selector3/1
  Initial state variable/1 -> Integration/2
  " "/1 -> Integration/1
  Bus Selector/1 -> " "/1  "<FCM(2;8)>"
  Bus Selector1/1 -> " "/2  "<FCM(2;9)>"
  Bus Selector2/1 -> " "/3  "<FCM(2;10)>"
  Bus Selector3/1 -> " "/4  "<FCM(2;11)>"
  Constant/1 -> Initial state variable/1

== system COSTEP/Separator/Holdup of Components in Separator/YP(12) ==
  FCM(3,8) : Inport
  FCM(3,9) : Inport  Port=2
  FCM(3,10) : Inport  Port=3
  FCM(3,11) : Inport  Port=4
  " " : Sum  Inputs=+---
  Bus Selector : BusSelector  OutputSignals=FCM(3;11)
  Bus Selector1 : BusSelector  OutputSignals=FCM(3;10)
  Bus Selector2 : BusSelector  OutputSignals=FCM(3;9)
  Bus Selector3 : BusSelector  OutputSignals=FCM(3;8)
  Constant : Constant  Value=12
  Initial state variable : mylib/Initial state variable
  Integration : mylib/Integration  SystemSampleTime=-1  VariantActivationTime=update diagram  AllowFlexibleInterface=on  Latency=0  AutoFrameSizeCalculation=off
  YY(12) : Outport  VectorParamsAs1DForOutWhenUnconnected=off
  wires:
  Integration/1 -> YY(12)/1
  FCM(3,8)/1 -> Bus Selector3/1
  FCM(3,9)/1 -> Bus Selector2/1
  FCM(3,10)/1 -> Bus Selector1/1
  FCM(3,11)/1 -> Bus Selector/1
  " "/1 -> Integration/1
  Initial state variable/1 -> Integration/2
  Bus Selector3/1 -> " "/1  "<FCM(3;8)>"
  Bus Selector2/1 -> " "/2  "<FCM(3;9)>"
  Bus Selector1/1 -> " "/3  "<FCM(3;10)>"
  Bus Selector/1 -> " "/4  "<FCM(3;11)>"
  Constant/1 -> Initial state variable/1

== system COSTEP/Separator/Holdup of Components in Separator/YP(13) ==
  FCM(4,8) : Inport
  FCM(4,9) : Inport  Port=2
  FCM(4,10) : Inport  Port=3
  FCM(4,11) : Inport  Port=4
  " " : Sum  Inputs=+---
  Bus Selector : BusSelector  OutputSignals=FCM(4;11)
  Bus Selector1 : BusSelector  OutputSignals=FCM(4;10)
  Bus Selector2 : BusSelector  OutputSignals=FCM(4;9)
  Bus Selector3 : BusSelector  OutputSignals=FCM(4;8)
  Constant : Constant  Value=13
  Initial state variable : mylib/Initial state variable
  Integration : mylib/Integration  SystemSampleTime=-1  VariantActivationTime=update diagram  AllowFlexibleInterface=on  Latency=0  AutoFrameSizeCalculation=off
  "YY(13) " : Outport  VectorParamsAs1DForOutWhenUnconnected=off
  wires:
  Integration/1 -> "YY(13) "/1
  FCM(4,8)/1 -> Bus Selector3/1
  FCM(4,9)/1 -> Bus Selector2/1
  FCM(4,10)/1 -> Bus Selector1/1
  FCM(4,11)/1 -> Bus Selector/1
  " "/1 -> Integration/1
  Initial state variable/1 -> Integration/2
  Bus Selector3/1 -> " "/1  "<FCM(4;8)>"
  Bus Selector2/1 -> " "/2  "<FCM(4;9)>"
  Bus Selector1/1 -> " "/3  "<FCM(4;10)>"
  Bus Selector/1 -> " "/4  "<FCM(4;11)>"
  Constant/1 -> Initial state variable/1

== system COSTEP/Separator/Holdup of Components in Separator/YP(14) ==
  FCM(5,8) : Inport
  FCM(5,9) : Inport  Port=2
  FCM(5,10) : Inport  Port=3
  FCM(5,11) : Inport  Port=4
  " " : Sum  Inputs=+---
  Bus Selector : BusSelector  OutputSignals=FCM(5;8)
  Bus Selector1 : BusSelector  OutputSignals=FCM(5;9)
  Bus Selector2 : BusSelector  OutputSignals=FCM(5;11)
  Bus Selector3 : BusSelector  OutputSignals=FCM(5;10)
  Constant : Constant  Value=14
  Initial state variable : mylib/Initial state variable
  Integration : mylib/Integration  SystemSampleTime=-1  VariantActivationTime=update diagram  AllowFlexibleInterface=on  Latency=0  AutoFrameSizeCalculation=off
  "YY(14) " : Outport  VectorParamsAs1DForOutWhenUnconnected=off
  wires:
  Integration/1 -> "YY(14) "/1
  FCM(5,8)/1 -> Bus Selector/1
  FCM(5,9)/1 -> Bus Selector1/1
  FCM(5,10)/1 -> Bus Selector3/1
  FCM(5,11)/1 -> Bus Selector2/1
  " "/1 -> Integration/1
  Initial state variable/1 -> Integration/2
  Bus Selector/1 -> " "/1  "<FCM(5;8)>"
  Bus Selector1/1 -> " "/2  "<FCM(5;9)>"
  Bus Selector3/1 -> " "/3  "<FCM(5;10)>"
  Bus Selector2/1 -> " "/4  "<FCM(5;11)>"
  Constant/1 -> Initial state variable/1

== system COSTEP/Separator/Holdup of Components in Separator/YP(15) ==
  FCM(6,8) : Inport
  FCM(6,9) : Inport  Port=2
  FCM(6,10) : Inport  Port=3
  FCM(6,11) : Inport  Port=4
  " " : Sum  Inputs=+---
  Bus Selector : BusSelector  OutputSignals=FCM(6;8)
  Bus Selector1 : BusSelector  OutputSignals=FCM(6;11)
  Bus Selector2 : BusSelector  OutputSignals=FCM(6;10)
  Bus Selector3 : BusSelector  OutputSignals=FCM(6;9)
  Constant : Constant  Value=15
  Initial state variable : mylib/Initial state variable
  Integration : mylib/Integration  SystemSampleTime=-1  VariantActivationTime=update diagram  AllowFlexibleInterface=on  Latency=0  AutoFrameSizeCalculation=off
  "YY(15) " : Outport  VectorParamsAs1DForOutWhenUnconnected=off
  wires:
  Integration/1 -> "YY(15) "/1
  FCM(6,8)/1 -> Bus Selector/1
  FCM(6,9)/1 -> Bus Selector3/1
  FCM(6,10)/1 -> Bus Selector2/1
  FCM(6,11)/1 -> Bus Selector1/1
  " "/1 -> Integration/1
  Initial state variable/1 -> Integration/2
  Bus Selector3/1 -> " "/2  "<FCM(6;9)>"
  Bus Selector2/1 -> " "/3  "<FCM(6;10)>"
  Bus Selector1/1 -> " "/4  "<FCM(6;11)>"
  Bus Selector/1 -> " "/1  "<FCM(6;8)>"
  Constant/1 -> Initial state variable/1

== system COSTEP/Separator/Holdup of Components in Separator/YP(16) ==
  FCM(7,8) : Inport
  FCM(7,9) : Inport  Port=2
  FCM(7,10) : Inport  Port=3
  FCM(7,11) : Inport  Port=4
  " " : Sum  Inputs=+---
  Bus Selector : BusSelector  OutputSignals=FCM(7;11)
  Bus Selector1 : BusSelector  OutputSignals=FCM(7;10)
  Bus Selector2 : BusSelector  OutputSignals=FCM(7;9)
  Bus Selector3 : BusSelector  OutputSignals=FCM(7;8)
  Constant : Constant  Value=16
  Initial state variable : mylib/Initial state variable
  Integration : mylib/Integration  SystemSampleTime=-1  VariantActivationTime=update diagram  AllowFlexibleInterface=on  Latency=0  AutoFrameSizeCalculation=off
  "YY(16) " : Outport  VectorParamsAs1DForOutWhenUnconnected=off
  wires:
  Integration/1 -> "YY(16) "/1
  FCM(7,8)/1 -> Bus Selector3/1
  FCM(7,9)/1 -> Bus Selector2/1
  FCM(7,10)/1 -> Bus Selector1/1
  FCM(7,11)/1 -> Bus Selector/1
  " "/1 -> Integration/1
  Initial state variable/1 -> Integration/2
  Bus Selector3/1 -> " "/1  "<FCM(7;8)>"
  Bus Selector2/1 -> " "/2  "<FCM(7;9)>"
  Bus Selector1/1 -> " "/3  "<FCM(7;10)>"
  Bus Selector/1 -> " "/4  "<FCM(7;11)>"
  Constant/1 -> Initial state variable/1

== system COSTEP/Separator/Holdup of Components in Separator/YP(17) ==
  FCM(8,8) : Inport
  FCM(8,9) : Inport  Port=2
  FCM(8,10) : Inport  Port=3
  FCM(8,11) : Inport  Port=4
  " " : Sum  Inputs=+---
  Bus Selector : BusSelector  OutputSignals=FCM(8;11)
  Bus Selector1 : BusSelector  OutputSignals=FCM(8;10)
  Bus Selector2 : BusSelector  OutputSignals=FCM(8;9)
  Bus Selector3 : BusSelector  OutputSignals=FCM(8;8)
  Constant : Constant  Value=17
  Initial state variable : mylib/Initial state variable
  Integration : mylib/Integration  SystemSampleTime=-1  VariantActivationTime=update diagram  AllowFlexibleInterface=on  Latency=0  AutoFrameSizeCalculation=off
  "YY(17) " : Outport  VectorParamsAs1DForOutWhenUnconnected=off
  wires:
  Integration/1 -> "YY(17) "/1
  FCM(8,8)/1 -> Bus Selector3/1
  FCM(8,9)/1 -> Bus Selector2/1
  FCM(8,10)/1 -> Bus Selector1/1
  " "/1 -> Integration/1
  Initial state variable/1 -> Integration/2
  FCM(8,11)/1 -> Bus Selector/1
  Bus Selector3/1 -> " "/1  "<FCM(8;8)>"
  Bus Selector2/1 -> " "/2  "<FCM(8;9)>"
  Bus Selector1/1 -> " "/3  "<FCM(8;10)>"
  Bus Selector/1 -> " "/4  "<FCM(8;11)>"
  Constant/1 -> Initial state variable/1

== system COSTEP/Separator/Pressure of Separator/Subsystem ==
  TCS : Inport
  VVS : Inport  Port=2
  UCVS : Inport  Port=3
  Bus Selector : BusSelector  OutputSignals=UCVS(1),UCVS(2),UCVS(3)
  PPS(1) Partial pressure of Component A mmHg : Product  Inputs=***/
  PPS(2) Partial pressure of Component B mmHg : Product  Inputs=***/
  PPS(3) Partial pressure of Component C mmHg : Product  Inputs=***/
  RG Universal Gas Constant ft³·mmHg/K·lb-mol : Constant  Value=998.9
  TKS Temperature in Separator K : Sum
  To Convert °C to K : Constant  Value=273.15
  PPS(1) : Outport  VectorParamsAs1DForOutWhenUnconnected=off
  PPS(2) : Outport  Port=2  VectorParamsAs1DForOutWhenUnconnected=off
  PPS(3) : Outport  Port=3  VectorParamsAs1DForOutWhenUnconnected=off
  wires:
  Bus Selector/3 -> PPS(3) Partial pressure of Component C mmHg/1  "<UCVS(3)>"
  RG Universal Gas Constant ft³·mmHg/K·lb-mol/1 -> PPS(3) Partial pressure of Component C mmHg/2, PPS(1) Partial pressure of Component A mmHg/2, PPS(2) Partial pressure of Component B mmHg/2
  UCVS/1 -> Bus Selector/1
  Bus Selector/1 -> PPS(1) Partial pressure of Component A mmHg/1  "<UCVS(1)>"
  Bus Selector/2 -> PPS(2) Partial pressure of Component B mmHg/1  "<UCVS(2)>"
  VVS/1 -> PPS(3) Partial pressure of Component C mmHg/4, PPS(2) Partial pressure of Component B mmHg/4, PPS(1) Partial pressure of Component A mmHg/4
  PPS(3) Partial pressure of Component C mmHg/1 -> PPS(3)/1
  To Convert °C to K/1 -> TKS Temperature in Separator K/2
  PPS(1) Partial pressure of Component A mmHg/1 -> PPS(1)/1
  TKS Temperature in Separator K/1 -> PPS(3) Partial pressure of Component C mmHg/3, PPS(2) Partial pressure of Component B mmHg/3, PPS(1) Partial pressure of Component A mmHg/3
  PPS(2) Partial pressure of Component B mmHg/1 -> PPS(2)/1
  TCS/1 -> TKS Temperature in Separator K/1

== system COSTEP/Separator/Pressure of Separator/VPR Vapour Pressure mmHg ==
  TCS : Inport
  AVP(I) Antoine Coefficient A ln(mmHg) : Constant  Value=AVP
  Add : Sum
  Add1 : Sum
  BVP(I) Antoine Coefficient B ln(mmHg)·°C : Constant  Value=BVP
  CVP(I) Antoine Coefficient C °C : Constant  Value=CVP
  Divide : Product  Inputs=*/
  Math Function : Math  SignedPower=on
  VPR : Outport  VectorParamsAs1DForOutWhenUnconnected=off
  wires:
  BVP(I) Antoine Coefficient B ln(mmHg)·°C/1 -> Divide/1
  CVP(I) Antoine Coefficient C °C/1 -> Add/1
  AVP(I) Antoine Coefficient A ln(mmHg)/1 -> Add1/1
  Add/1 -> Divide/2
  Divide/1 -> Add1/2
  Add1/1 -> Math Function/1
  Math Function/1 -> VPR/1
  TCS/1 -> Add/2

== system COSTEP/Separator/Stream 10/HST(10) Molar Enthalpy of Stream 10 MBtu//lb-mol ==
  ITY : Inport
  T : Inport  Port=2
  XST(I,I) : Inport  Port=3
  "Enthalpy of Stream " : mylib/Enthalpy of Stream   SystemSampleTime=-1  VariantActivationTime=update diagram  AllowFlexibleInterface=on  Latency=0  AutoFrameSizeCalculation=off
  "H " : Outport  VectorParamsAs1DForOutWhenUnconnected=off
  wires:
  ITY/1 -> "Enthalpy of Stream "/1
  T/1 -> "Enthalpy of Stream "/2
  XST(I,I)/1 -> "Enthalpy of Stream "/3
  "Enthalpy of Stream "/1 -> "H "/1

== system COSTEP/Separator/Stream 10/Subsystem ==
  VPOS(6) : Inport  PortDimensions=1
  Abs : Abs  SaturateOnIntegerOverflow=off
  Constant : Constant  Value=0.0
  Constant1 : Constant  Value=0.151169
  Constant2 : Constant  Value=760
  DLP : Sum  Inputs=+-
  DLP Pressure drop between separator and environment : Merge
  FLMS : Product  Inputs=3
  If : If  IfExpression=u1 < 0
  If Action Subsystem : Subsystem  TreatAsAtomicUnit=on
  If Action Subsystem1 : Subsystem  TreatAsAtomicUnit=on
  Sqrt : Sqrt
  Out1 : Outport  VectorParamsAs1DForOutWhenUnconnected=off
  wires:
  Constant2/1 -> DLP/2
  Constant1/1 -> FLMS/2
  Abs/1 -> Sqrt/1
  DLP Pressure drop between separator and environment/1 -> Abs/1
  [PTS] -> DLP/1
  If Action Subsystem/1(Out1) -> DLP Pressure drop between separator and environment/1
  Constant/1 -> If Action Subsystem/1(In1)
  Sqrt/1 -> FLMS/3
  If Action Subsystem1/1(Out1) -> DLP Pressure drop between separator and environment/2
  If/2 -> If Action Subsystem1/Action
  DLP/1 -> If Action Subsystem1/1(In1), If/1
  VPOS(6)/1 -> FLMS/1
  If/1 -> If Action Subsystem/Action
  FLMS/1 -> Out1/1

== system COSTEP/Separator/Stream 10/XMWS(10) Molecular weight of Stream 10 lb//lb-mol ==
  XST(I,10) : Inport
  Constant : Constant  Value=XMW
  Product : Product
  Sum of Elements : Sum  Inputs=+
  XMWS(10) : Outport  VectorParamsAs1DForOutWhenUnconnected=off
  wires:
  Sum of Elements/1 -> XMWS(10)/1
  Product/1 -> Sum of Elements/1
  XST(I,10)/1 -> Product/1
  Constant/1 -> Product/2
